simulink model "Model"  (R2024b)
settings: Solver=VariableStepAuto  StartTime=0.0  StopTime=5  RelTol=1e-3
undefined symbols (not defined in the file or in its folder): beta_eq, Jeq, Jm_rotor, km, Lm, Rm
settings Model: Creator=Student  LastModifiedBy=Student

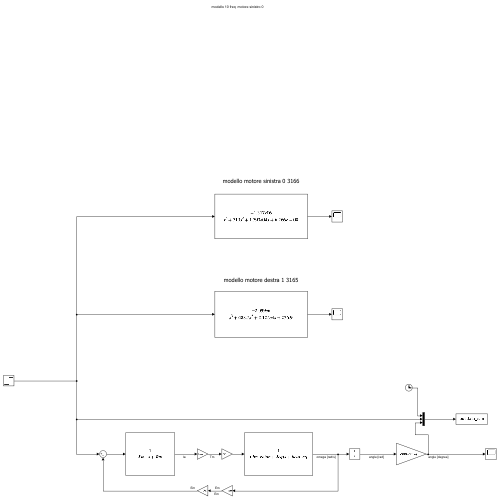
[thumbnail: Simulink's stored preview of the top-level diagram]
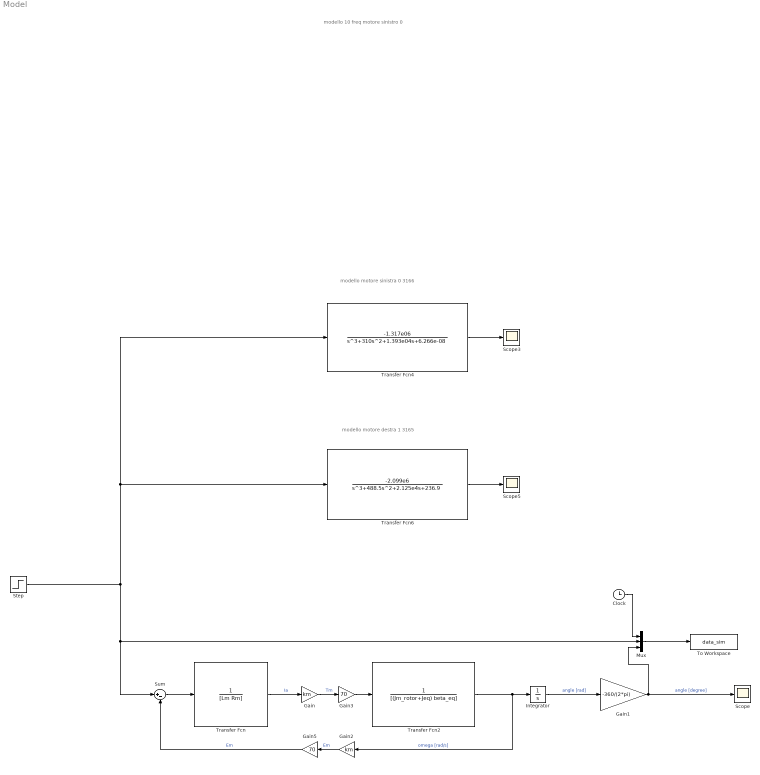
== system Model ==
  note: modello motore sinistra 0 3166
  note: modello 10 freq motore sinistro 0
  note: modello motore destra 1 3165
  Clock : Clock
  Gain : Gain  Gain=km
  Gain1 : Gain  Gain=-360/(2*pi)
  Gain2 : Gain  Gain=km
  Gain3 : Gain  Gain=70
  Gain5 : Gain  Gain=70
  Integrator : Integrator
  Mux : Mux  Inputs=3
  Scope : Scope
  Scope3 : Scope
  Scope5 : Scope
  Step : Step  SampleTime=0
  Sum : Sum  Inputs=|+-
  To Workspace : ToWorkspace  VariableName=data_sim  SampleTime=0.002
  Transfer Fcn : TransferFcn  Denominator=[Lm Rm]
  Transfer Fcn2 : TransferFcn  Denominator=[(Jm_rotor+Jeq) beta_eq]
  Transfer Fcn4 : TransferFcn  Numerator=[-1.317e06]  Denominator=[1 310 1.393e04 6.266e-08]
  Transfer Fcn6 : TransferFcn  Numerator=[-2.099e6]  Denominator=[1 488.5 2.125e4 236.9]
  wires:
  Transfer Fcn/1 -> Gain/1  "Ia"
  Transfer Fcn2/1 -> Gain2/1, Integrator/1  "omega [rad/s]"
  Integrator/1 -> Gain1/1  "angle [rad]"
  Sum/1 -> Transfer Fcn/1
  Gain2/1 -> Gain5/1  "Em"
  Gain1/1 -> Mux/3, Scope/1  "angle [degree]"
  Gain3/1 -> Transfer Fcn2/1
  Gain/1 -> Gain3/1  "Tm"
  Gain5/1 -> Sum/2  "Em"
  Step/1 -> Transfer Fcn4/1, Transfer Fcn6/1, Mux/2, Sum/1
  Mux/1 -> To Workspace/1
  Clock/1 -> Mux/1
  Transfer Fcn4/1 -> Scope3/1
  Transfer Fcn6/1 -> Scope5/1
